simulink model "Prob_4"  (R2020b)
settings: Solver=VariableStepAuto  StartTime=0.0  StopTime=0.01  RelTol=1e-3
undefined symbols (not defined in the file or in its folder): b, J, K, L, R
settings Model: DataDictionary=W2_Prob4.sldd  Creator=kshir  LastModifiedBy=kshir

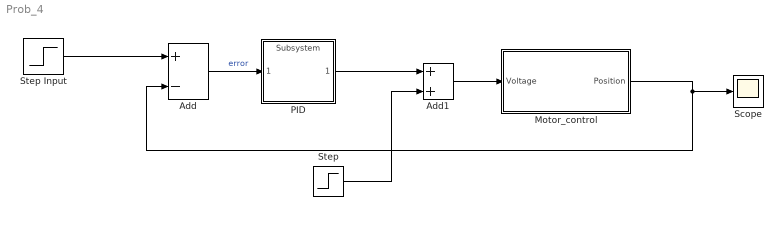
== system Prob_4 ==
  Add : Sum  Inputs=+-
  Add1 : Sum
  Motor_control : Subsystem
  PID : ModelReference  ModelNameDialog=Subsystem  SimulationMode=Normal  ModelReferenceVersion=1.3
  Scope : Scope
  Step : Step  Time=0  SampleTime=0
  Step Input : Step  Time=0  SampleTime=0
  wires:
  Add/1 -> PID/1  "error"
  Step Input/1 -> Add/1
  Motor_control/1(Position) -> Add/2, Scope/1
  PID/1 -> Add1/1
  Add1/1 -> Motor_control/1(Voltage)
  Step/1 -> Add1/2

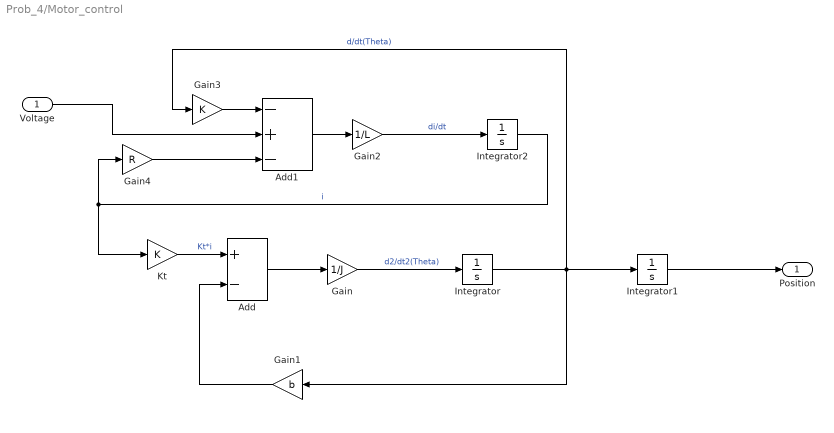
== system Prob_4/Motor_control ==
  Voltage : Inport
  Add : Sum  Inputs=+-
  Add1 : Sum  Inputs=-+-
  Gain : Gain  Gain=1/J
  Gain1 : Gain  Gain=b
  Gain2 : Gain  Gain=1/L
  Gain3 : Gain  Gain=K
  Gain4 : Gain  Gain=R
  Integrator : Integrator
  Integrator1 : Integrator
  Integrator2 : Integrator
  Kt : Gain  Gain=K
  Position : Outport
  wires:
  Gain1/1 -> Add/2
  Integrator2/1 -> Gain4/1, Kt/1  "i"
  Add/1 -> Gain/1
  Integrator/1 -> Gain3/1, Gain1/1, Integrator1/1  "d/dt(Theta)"
  Gain3/1 -> Add1/1
  Gain/1 -> Integrator/1  "d2/dt2(Theta)"
  Gain4/1 -> Add1/3
  Add1/1 -> Gain2/1
  Kt/1 -> Add/1  "Kt*i"
  Gain2/1 -> Integrator2/1  "di/dt"
  Voltage/1 -> Add1/2
  Integrator1/1 -> Position/1
